simulink model "danxiangtiaoya"  (R2019b)
settings: Solver=ode15s  StartTime=0.0  StopTime=0.04  RelTol=1e-3  EnableMultiTasking=on
libraries: powerlib x8
settings Model: Creator=Administrator  LastModifiedBy=bhisma
settings DataIOCC: LimitDataPoints=on  SaveFormat=Array  SignalLoggingSaveFormat=ModelDataLogs  SaveOutput=off  SaveTime=off  ReturnWorkspaceOutputs=off
settings OptimizationCC: BooleanDataType=off  InitFltsAndDblsToZero=on  LifeSpan=inf
settings DebuggingCC: SaveWithParameterizedLinksMsg=none  UnderspecifiedInitializationDetection=Classic  MergeDetectMultiDrivingBlocksExec=none  SignalResolutionControl=TryResolveAllWithWarning  MultiTaskDSMMsg=warning  MultiTaskCondExecSysMsg=none  FcnCallInpInsideContextMsg=warning  AllowSymbolicDim=off  SFUnexpectedBacktrackingDiag=warning  SFNoUnconditionalDefaultTransitionDiag=warning  SFExecutionAtInitializationDiag=none  ArithmeticOperatorsInVariantConditions=warning
settings HardwareCC: ProdBitPerPointer=32  ProdBitPerSizeT=32  ProdBitPerPtrDiffT=32  ProdLargestAtomicFloat=None  ProdIntDivRoundTo=Undefined  ProdEndianess=Unspecified  ProdWordSize=32  ProdHWDeviceType=32-bit Generic  TargetUnknown=on
settings ModelReferenceCC: PropagateSignalLabelsOutOfModel=off
settings SFSimCC: SimUseLocalCustomCode=off  CustomCodeUndefinedFunction=UseInterfaceOnly
settings RTWCC: RTWUseLocalCustomCode=off
settings CodeAppCC: StateflowObjectComments=on
settings GRTTargetCC: TargetFcnLib=ansi_tfl_tmw.mat  TargetLangStandard=C89/C90 (ANSI)  CombineOutputUpdateFcns=off  GRTInterface=on
settings ConfigComp: CovMetricSettings=dw  CovHtmlReporting=on  CovSaveCumulativeToWorkspaceVar=on  CovSaveSingleToWorkspaceVar=on  CovExternalEMLEnable=off
settings SimscapeCC: SimscapeNormalizeSystem=off

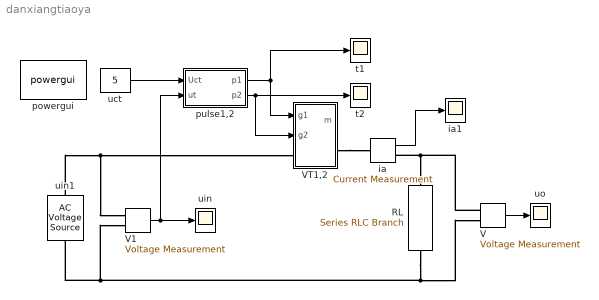
== system danxiangtiaoya ==
  RL : powerlib/Elements/Series RLC Branch  LConnTagsString=__new0  RConnTagsString=__new0  BranchType=RL  Resistance=1  Inductance=1e-3  SetiL0=off  InitialCurrent=0  Capacitance=[]  Setx0=off  InitialVoltage=0  Measurements=None
      settings: SourceProductName=Simscape Electrical
  V : powerlib/Measurements/Voltage Measurement  PhasorSimulation=off  OutputType=Magnitude  PSBequivalent=0
      settings: SourceProductName=Simscape Electrical
  V1 : powerlib/Measurements/Voltage Measurement  PhasorSimulation=off  OutputType=Magnitude  PSBequivalent=0
      settings: SourceProductName=Simscape Electrical
  VT1,2 : Subsystem
  ia : powerlib/Measurements/Current Measurement  PhasorSimulation=off  OutputType=Magnitude  PSBequivalent=0
      settings: SourceProductName=Simscape Electrical
  ia1 : Scope
  powergui : powerlib/powergui  Priority=1  SimulationMode=Continuous  SampleTime=50e-6  frequency=60  Iterations=50  frequencyindice=50  Pbase=100e6  ErrMax=1e-4  UnitsV=kV  UnitsW=MW  buscounter=0  FunctionMessages=off  echomessages=off  EnableUseOfTLC=off  CurrentSourceSwitches=off  DisableSnubberDevices=off  DisableRonSwitches=off  DisableVfSwitches=off  DisplayEquations=off  AutomaticDiscreteSolvers=off  SolverType=Tustin/Backward Euler (TBE)  Interpol=off  ExternalGateDelay=off  methode=off  Ts=10  x0status=blocks  SPID=off  SwTol=0  HookPort=off  NonlinearTolerance=1e-4  nMaxIteration=100  ContinueOnMaxIteration=off  RestoreLinks=warning  ResistiveCurrentMeasurement=off  Frange=[0:2:500]  Ylog=off  Xlog=on  ShowGrid=off  save=off  variable=ZData  structure=0  ZoomFFT=off  StartTime=0.0  cycles=1  DisplayStyle=1  fundamental=60  FreqAxis=off  MaxFrequency=1000  frequencyindicesteady=1  RmsSteady=1  display=off
      settings: SourceProductName=Simscape Electrical
  pulse1,2 : Subsystem
  t1 : Scope
  t2 : Scope
  uct : Constant  Value=5
  uin : Scope
  uin1 : powerlib/Electrical Sources/AC Voltage Source  Amplitude=220  Phase=0  Frequency=50  SampleTime=0  Measurements=None  BusType=swing  Pref=10e3  Qref=0  Qmin=-inf  Qmax=+inf
      settings: SourceProductName=Simscape Electrical
  uo : Scope
  wires:
  V/1 -> uo/1
  ia/1 -> ia1/1
  pulse1,2/1(p1) -> t1/1, VT1,2/1(g1)
  pulse1,2/2(p2) -> t2/1, VT1,2/2(g2)
  uct/1 -> pulse1,2/1(Uct)
  V1/1 -> uin/1, pulse1,2/2(ut)
  connections:
  uin1/RConn1 -- VT1,2/LConn1 -- V1/LConn1
  RL/RConn1 -- V/LConn2 -- uin1/LConn1 -- V1/LConn2
  V/LConn1 -- ia/RConn1 -- RL/LConn1
  VT1,2/RConn1 -- ia/LConn1

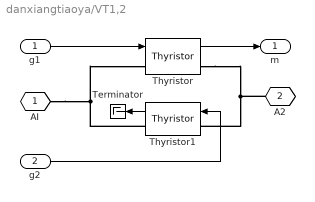
== system danxiangtiaoya/VT1,2 ==
  g1 : Inport
  g2 : Inport  Port=2
  Terminator : Terminator
  Thyristor : powerlib/Power Electronics/Thyristor  Ron=1e-03  Lon=0  Vf=0.8  IC=0  Rs=1000  Cs=inf  Measurements=on
      settings: SourceProductName=Simscape Electrical
  Thyristor1 : powerlib/Power Electronics/Thyristor  Ron=1e-03  Lon=0  Vf=0.8  IC=0  Rs=1000  Cs=inf  Measurements=on
      settings: SourceProductName=Simscape Electrical
  AI : PMIOPort  Tag=PMCPort  Side=Left
  A2 : PMIOPort  Tag=PMCPort  Port=2  Side=Right
  m : Outport
  wires:
  g1/1 -> Thyristor/1
  g2/1 -> Thyristor1/1
  Thyristor/1 -> m/1
  Thyristor1/1 -> Terminator/1
  connections:
  Thyristor1/RConn1 -- Thyristor/LConn1 -- AI/RConn1
  Thyristor/RConn1 -- Thyristor1/LConn1 -- A2/RConn1

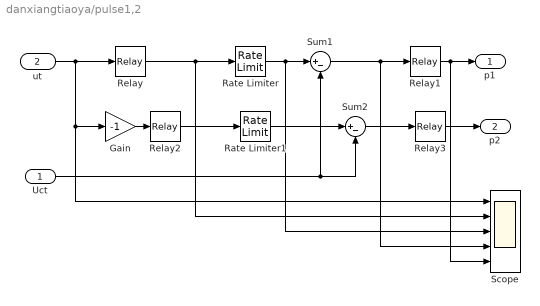
== system danxiangtiaoya/pulse1,2 ==
  Uct : Inport
  ut : Inport  Port=2
  Gain : Gain  Gain=-1  SaturateOnIntegerOverflow=on  OutDataTypeStr=Inherit: Same as input  ParamDataTypeStr=Inherit: Same as input
  Rate Limiter : RateLimiter  RisingSlewLimit=1000  FallingSlewLimit=-1e8
  Rate Limiter1 : RateLimiter  RisingSlewLimit=1000  FallingSlewLimit=-1e8
  Relay : Relay  OnOutputValue=10
  Relay1 : Relay
  Relay2 : Relay  OnOutputValue=10
  Relay3 : Relay
  Scope : Scope  NumInputPorts=5
  Sum1 : Sum  Inputs=|+-  SaturateOnIntegerOverflow=on  InputSameDT=on  OutDataTypeStr=Inherit: Same as first input
  Sum2 : Sum  Inputs=|+-  SaturateOnIntegerOverflow=on  InputSameDT=on  OutDataTypeStr=Inherit: Same as first input
  p1 : Outport
  p2 : Outport  Port=2
  wires:
  Relay/1 -> Rate Limiter/1, Scope/2
  Rate Limiter/1 -> Sum1/1, Scope/3
  Sum1/1 -> Relay1/1, Scope/4
  Gain/1 -> Relay2/1
  Rate Limiter1/1 -> Sum2/1
  Sum2/1 -> Relay3/1
  Relay2/1 -> Rate Limiter1/1
  Relay1/1 -> p1/1, Scope/5
  Relay3/1 -> p2/1
  ut/1 -> Relay/1, Gain/1, Scope/1
  Uct/1 -> Sum2/2, Sum1/2
